simulink model "Observer_mode_model2"  (R2024a)
settings: Solver=VariableStepAuto  StartTime=0.0  StopTime=10.0  RelTol=1e-3
undefined symbols (not defined in the file or in its folder): Hecate_time, Hecate_u1, Hecate_u2, Hecate_u3, Hecate_u4
settings Model: Creator=The MathWorks, Inc.  LastModifiedBy=fedformi_new
settings SolverCC: MaxZcPerStep=1
settings OptimizationCC: ReuseModelBlockBuffer=off
settings DebuggingCC: UnconnectedInputMsg=warning  UnconnectedOutputMsg=warning  UnconnectedLineMsg=warning
settings ModelReferenceCC: EnableRefExpFcnMdlSchedulingChecks=on
settings RTWCC: GPUComputeCapability=3.5  DLArmComputeVersion=19.05

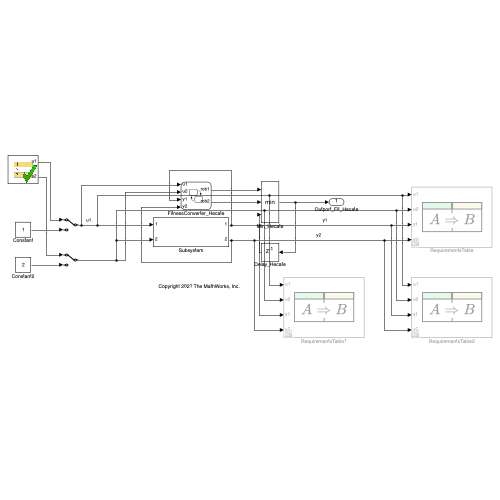
[thumbnail: Simulink's stored preview of the top-level diagram]
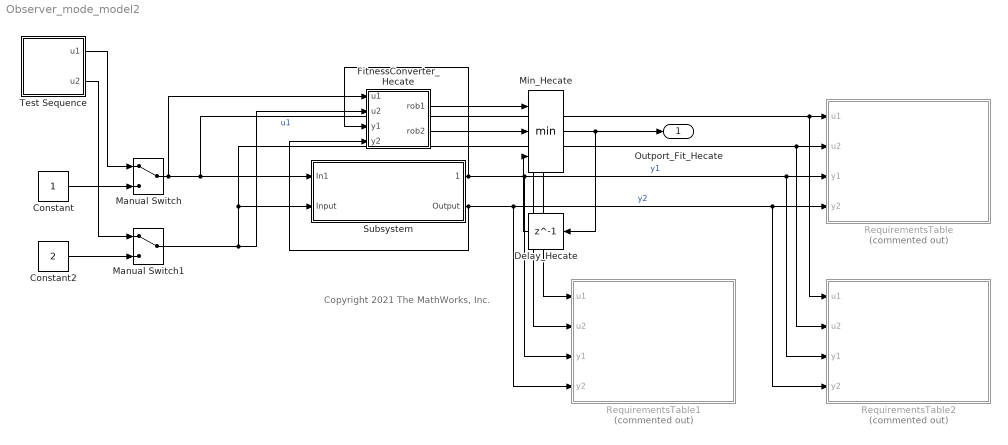
== system Observer_mode_model2 ==
  note: Copyright 2021 The MathWorks, Inc.
  Constant : Constant
  Constant2 : Constant  Value=2
  Delay_Hecate : Delay  DelayLength=1  InitialCondition=Inf
  FitnessConverter_Hecate : Stateflow chart  TreatAsAtomicUnit=on
  Manual Switch : ManualSwitch
  Manual Switch1 : ManualSwitch
  Min_Hecate : MinMax  Inputs=3
  RequirementsTable : Requirements Table  Commented=on  TreatAsAtomicUnit=on
  RequirementsTable1 : Requirements Table  Commented=on  TreatAsAtomicUnit=on
  RequirementsTable2 : Requirements Table  Commented=on  TreatAsAtomicUnit=on
  Subsystem : Subsystem
  Test Sequence : Test Sequence  TreatAsAtomicUnit=on
  Outport_Fit_Hecate : Outport
  wires:
  Subsystem/2(Output) -> RequirementsTable1/4(y2), RequirementsTable2/4(y2), RequirementsTable/4(y2), FitnessConverter_Hecate/4(y2)  "y2"
  Manual Switch/1 -> Subsystem/1(In1), RequirementsTable1/1(u1), RequirementsTable2/1(u1), RequirementsTable/1(u1), FitnessConverter_Hecate/1(u1)  "u1"
  Manual Switch1/1 -> Subsystem/2(Input), RequirementsTable1/2(u2), RequirementsTable2/2(u2), RequirementsTable/2(u2), FitnessConverter_Hecate/2(u2)
  Subsystem/1(1) -> RequirementsTable1/3(y1), RequirementsTable2/3(y1), RequirementsTable/3(y1), FitnessConverter_Hecate/3(y1)  "y1"
  Constant/1 -> Manual Switch/2
  Constant2/1 -> Manual Switch1/2
  Test Sequence/1(u1) -> Manual Switch/1
  Test Sequence/2(u2) -> Manual Switch1/1
  FitnessConverter_Hecate/1(rob1) -> Min_Hecate/1
  FitnessConverter_Hecate/2(rob2) -> Min_Hecate/2
  Min_Hecate/1 -> Delay_Hecate/1, Outport_Fit_Hecate/1
  Delay_Hecate/1 -> Min_Hecate/3

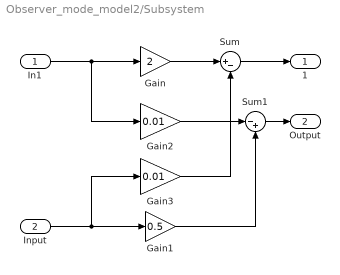
== system Observer_mode_model2/Subsystem ==
  In1 : Inport
  Input : Inport  Port=2
  Gain : Gain  Gain=2
  Gain1 : Gain  Gain=0.5
  Gain2 : Gain  Gain=0.01
  Gain3 : Gain  Gain=0.01
  Sum : Sum  Inputs=|+-
  Sum1 : Sum  Inputs=|-+
  1 : Outport
  Output : Outport  Port=2
  wires:
  In1/1 -> Gain2/1, Gain/1
  Input/1 -> Gain3/1, Gain1/1
  Gain1/1 -> Sum1/2
  Gain2/1 -> Sum1/1
  Gain/1 -> Sum/1
  Sum/1 -> 1/1
  Gain3/1 -> Sum/2
  Sum1/1 -> Output/1

== stateflow chart Observer_mode_model2/RequirementsTable1 ==
  (default) -> (junction 1073742836)
  (junction 1073742836) -> (junction 1073742837) : {
      | % SF_REQ_REV_07
      | }
  (junction 1073742837) -> (junction 1073742839) : {
      | % ExcEvals:
      | % PriEvals:
      | }
  (junction 1073742839) -> (junction 1073742841) : {
      | % HEADER_ASSIGNMENTS
      |
      | }
  (junction 1073742841) -> (junction 1073742843) : {
      | % START_A_4
      | }
  (junction 1073742843) -> (junction 1073742845) : {
      | }
  (junction 1073742845) -> (junction 1073742847)
  (junction 1073742847) -> (junction 1073742849) : {
      | }
  (junction 1073742849) -> (junction 1073742851) : {
      | % END_A_4
      | }
  (junction 1073742851) -> (junction 1073742853) : {
      | % START_R_7
      | }
  (junction 1073742853) -> (junction 1073742855) : {
      | }
  (junction 1073742855) -> (junction 1073742857)
  (junction 1073742857) -> (junction 1073742859) [order 1] : [(u1 > 0)]
  (junction 1073742857) -> (junction 1073742865) [order 2]
  (junction 1073742859) -> (junction 1073742861) : {
      | reqtable_postcondition((y1 > - 0.5), 'R:1');
      |
      |
      | }
  (junction 1073742861) -> (junction 1073742863) : {
      | }
  (junction 1073742863) -> (junction 1073742865)
  (junction 1073742865) -> (junction 1073742867)
  (junction 1073742867) -> (junction 1073742869) : {
      | % END_R_7
      | }
  (junction 1073742869) -> (junction 1073742871) : {
      | % START_R_1
      | }
  (junction 1073742871) -> (junction 1073742873) : {
      | }
  (junction 1073742873) -> (junction 1073742875)
  (junction 1073742875) -> (junction 1073742877) [order 1] : [(u2 > 0)]
  (junction 1073742875) -> (junction 1073742883) [order 2]
  (junction 1073742877) -> (junction 1073742879) : {
      | reqtable_postcondition((y2 > - 0.5), 'R:2');
      |
      |
      | }
  (junction 1073742879) -> (junction 1073742881) : {
      | }
  (junction 1073742881) -> (junction 1073742883)
  (junction 1073742883) -> (junction 1073742885)
  (junction 1073742885) -> (junction 1073742887) : {
      | % END_R_1
      | }
  (junction 1073742887) -> (junction 1073742889) : {
      | % START_R_10
      | }
  (junction 1073742889) -> (junction 1073742891) : {
      | }
  (junction 1073742891) -> (junction 1073742893) : {
      | reqtable_postcondition((0 < y1 || 0 >= y1 || 0 < y2 || 0 >= y2 ), 'R:3');
      |
      |
      | }
  (junction 1073742893) -> (junction 1073742895) : {
      | }
  (junction 1073742895) -> (junction 1073742897) : {
      | % END_R_10
      | }
  data: u1 input; u2 input; y1 input; y2 input

== stateflow chart Observer_mode_model2/RequirementsTable2 ==
  (default) -> (junction 1073742836)
  (junction 1073742836) -> (junction 1073742837) : {
      | % SF_REQ_REV_07
      | }
  (junction 1073742837) -> (junction 1073742839) : {
      | % ExcEvals:
      | % PriEvals:
      | }
  (junction 1073742839) -> (junction 1073742841) : {
      | % HEADER_ASSIGNMENTS
      |
      | }
  (junction 1073742841) -> (junction 1073742843) : {
      | % START_A_4
      | }
  (junction 1073742843) -> (junction 1073742845) : {
      | }
  (junction 1073742845) -> (junction 1073742847)
  (junction 1073742847) -> (junction 1073742849) : {
      | }
  (junction 1073742849) -> (junction 1073742851) : {
      | % END_A_4
      | }
  (junction 1073742851) -> (junction 1073742853) : {
      | % START_R_7
      | }
  (junction 1073742853) -> (junction 1073742855) : {
      | }
  (junction 1073742855) -> (junction 1073742857)
  (junction 1073742857) -> (junction 1073742859) [order 1] : [(u1 > - 0.5)]
  (junction 1073742857) -> (junction 1073742865) [order 2]
  (junction 1073742859) -> (junction 1073742861) : {
      | reqtable_postcondition((y1 > 0), 'R:1');
      |
      |
      | }
  (junction 1073742861) -> (junction 1073742863) : {
      | }
  (junction 1073742863) -> (junction 1073742865)
  (junction 1073742865) -> (junction 1073742867)
  (junction 1073742867) -> (junction 1073742869) : {
      | % END_R_7
      | }
  (junction 1073742869) -> (junction 1073742871) : {
      | % START_R_1
      | }
  (junction 1073742871) -> (junction 1073742873) : {
      | }
  (junction 1073742873) -> (junction 1073742875)
  (junction 1073742875) -> (junction 1073742877) [order 1] : [(u2 > - 0.5)]
  (junction 1073742875) -> (junction 1073742883) [order 2]
  (junction 1073742877) -> (junction 1073742879) : {
      | reqtable_postcondition((y2 > 0), 'R:2');
      |
      |
      | }
  (junction 1073742879) -> (junction 1073742881) : {
      | }
  (junction 1073742881) -> (junction 1073742883)
  (junction 1073742883) -> (junction 1073742885)
  (junction 1073742885) -> (junction 1073742887) : {
      | % END_R_1
      | }
  (junction 1073742887) -> (junction 1073742889) : {
      | % START_R_10
      | }
  (junction 1073742889) -> (junction 1073742891) : {
      | }
  (junction 1073742891) -> (junction 1073742893) : {
      | reqtable_postcondition((0 < y1 || 0 >= y1 || 0 < y2 || 0 >= y2 ), 'R:3');
      |
      |
      | }
  (junction 1073742893) -> (junction 1073742895) : {
      | }
  (junction 1073742895) -> (junction 1073742897) : {
      | % END_R_10
      | }
  data: u1 input; u2 input; y1 input; y2 input

== stateflow chart Observer_mode_model2/RequirementsTable ==
  (default) -> (junction 1073742836)
  (junction 1073742836) -> (junction 1073742837) : {
      | % SF_REQ_REV_07
      | }
  (junction 1073742837) -> (junction 1073742839) : {
      | % ExcEvals:
      | % PriEvals:
      | }
  (junction 1073742839) -> (junction 1073742841) : {
      | % HEADER_ASSIGNMENTS
      |
      | }
  (junction 1073742841) -> (junction 1073742843) : {
      | % START_A_4
      | }
  (junction 1073742843) -> (junction 1073742845) : {
      | }
  (junction 1073742845) -> (junction 1073742847)
  (junction 1073742847) -> (junction 1073742849) : {
      | }
  (junction 1073742849) -> (junction 1073742851) : {
      | % END_A_4
      | }
  (junction 1073742851) -> (junction 1073742853) : {
      | % START_R_7
      | }
  (junction 1073742853) -> (junction 1073742855) : {
      | }
  (junction 1073742855) -> (junction 1073742857)
  (junction 1073742857) -> (junction 1073742859) [order 1] : [(u1 > 0)]
  (junction 1073742857) -> (junction 1073742865) [order 2]
  (junction 1073742859) -> (junction 1073742861) : {
      | reqtable_postcondition((y1 > 0), 'R:1');
      |
      |
      | }
  (junction 1073742861) -> (junction 1073742863) : {
      | }
  (junction 1073742863) -> (junction 1073742865)
  (junction 1073742865) -> (junction 1073742867)
  (junction 1073742867) -> (junction 1073742869) : {
      | % END_R_7
      | }
  (junction 1073742869) -> (junction 1073742871) : {
      | % START_R_1
      | }
  (junction 1073742871) -> (junction 1073742873) : {
      | }
  (junction 1073742873) -> (junction 1073742875)
  (junction 1073742875) -> (junction 1073742877) [order 1] : [(u2 > 0)]
  (junction 1073742875) -> (junction 1073742883) [order 2]
  (junction 1073742877) -> (junction 1073742879) : {
      | reqtable_postcondition((y2 > 0), 'R:2');
      |
      |
      | }
  (junction 1073742879) -> (junction 1073742881) : {
      | }
  (junction 1073742881) -> (junction 1073742883)
  (junction 1073742883) -> (junction 1073742885)
  (junction 1073742885) -> (junction 1073742887) : {
      | % END_R_1
      | }
  (junction 1073742887) -> (junction 1073742889) : {
      | % START_R_10
      | }
  (junction 1073742889) -> (junction 1073742891) : {
      | }
  (junction 1073742891) -> (junction 1073742893) : {
      | reqtable_postcondition((0 < y1 || 0 >= y1 || 0 < y2 || 0 >= y2 ), 'R:3');
      |
      |
      | }
  (junction 1073742893) -> (junction 1073742895) : {
      | }
  (junction 1073742895) -> (junction 1073742897) : {
      | % END_R_10
      | }
  data: u1 input; u2 input; y1 input; y2 input

== stateflow chart Observer_mode_model2/Test Sequence ==
  state step_1
    u1 = Hecate_u1;
    u2 = Hecate_u2;
  state step_2
    u1 = Hecate_u3;
    u2 = Hecate_u4;
  (default) -> step_1
  step_1 -> step_2 : [
      | t >= Hecate_time
      | ]
  data: u1 output; u2 output; Hecate_u1 parameter; Hecate_u2 parameter; Hecate_u3 parameter; Hecate_u4 parameter; Hecate_time parameter

== stateflow chart Observer_mode_model2/FitnessConverter_Hecate ==
  state Requirement_1 [parallel]
    settings: executionOrder=1
    state Default
      rob1 = Inf;
    state Verify
      rob1 = (y1-(-0.5));
    (default) -> (junction 8)
    (junction 8) -> Requirement_1.Verify [order 2]
    (junction 8) -> Requirement_1.Default [order 1] : [~((u1>0))]
    Requirement_1.Default -> Requirement_1.Verify : [(u1>0)]
    Requirement_1.Verify -> Requirement_1.Default : [~((u1>0))]
  state Requirement_2 [parallel]
    settings: executionOrder=2
    state Default
      rob2 = Inf;
    state Verify
      rob2 = (y2-(-0.5));
    (default) -> (junction 17)
    (junction 17) -> Requirement_2.Verify [order 2]
    (junction 17) -> Requirement_2.Default [order 1] : [~((u2>0))]
    Requirement_2.Default -> Requirement_2.Verify : [(u2>0)]
    Requirement_2.Verify -> Requirement_2.Default : [~((u2>0))]
  data: u1 input; u2 input; y1 input; y2 input; rob1 output double =Inf; rob2 output double =Inf
